simulink model "foc_demo"  (R2021b)
settings: Solver=VariableStepAuto  StartTime=0.0  StopTime=1.0  RelTol=1e-3
undefined symbols (not defined in the file): Ki_cd, Ki_cq, Ki_w, Kp_cd, Kp_cq, Kp_w
libraries: slpidlib x3, spsDCVoltageSourceLib x1, spsPermanentMagnetSynchronousMachineLib x1, simulink x1, spsUniversalBridgeLib x1, spspowerguiLib x1
settings Model: SimulationMode=accelerator  Creator=Jiaxin Qian  LastModifiedBy=Jiaxin Qian

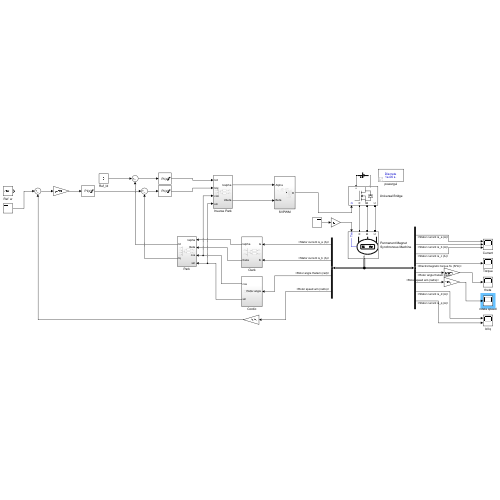
[thumbnail: Simulink's stored preview of the top-level diagram]
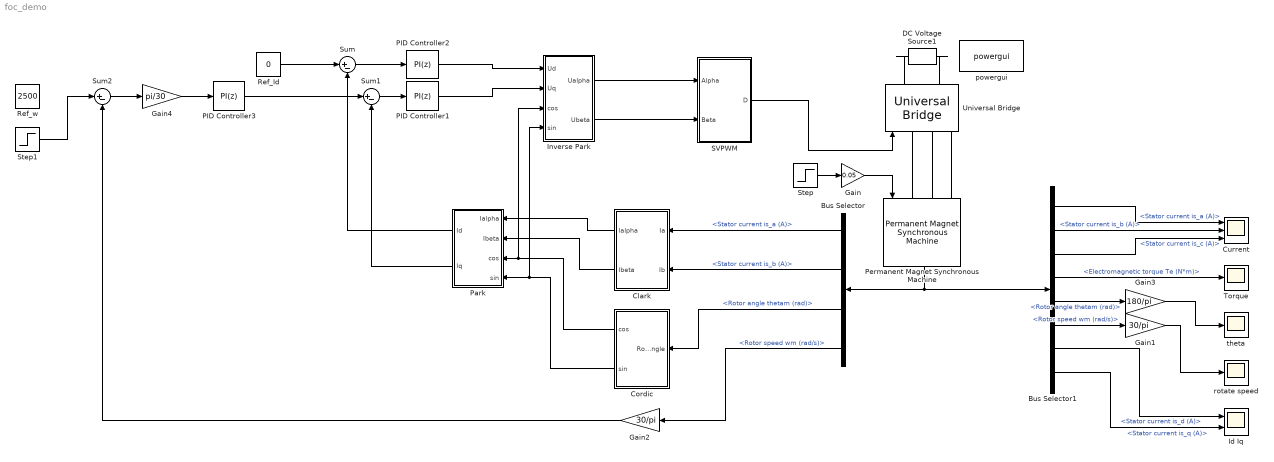
== system foc_demo ==
  Bus Selector : BusSelector  OutputSignals=Stator current is_a (A),Stator current is_b (A),Rotor angle thetam (rad),Rotor speed wm (rad/s)
  Bus Selector1 : BusSelector  OutputSignals=Stator current is_a (A),Stator current is_b (A),Stator current is_c (A),Electromagnetic torque Te (N*m),Rotor angle thetam (rad),Rotor speed wm (rad/s),Stator current is_d (A),Stator current is_q (A)
  Clark : Subsystem
  Cordic : Subsystem
  Current : Scope  NumInputPorts=3
  DC Voltage Source1 : spsDCVoltageSourceLib/DC Voltage Source  Amplitude=48  Measurements=None
  Gain : Gain  Gain=0.05
  Gain1 : Gain  Gain=30/pi
  Gain2 : Gain  Gain=30/pi
  Gain3 : Gain  Gain=180/pi
  Gain4 : Gain  Gain=pi/30
  Id Iq : Scope  NumInputPorts=2
  Inverse Park : Subsystem
  PID Controller1 : slpidlib/PID Controller  Controller=PI  Form=Parallel  TimeDomain=Discrete-time  UseExternalTs=off  SampleTime=-1  IntegratorMethod=Forward Euler  FilterMethod=Forward Euler  ControllerParametersSource=internal  P=Kp_cq  I=Ki_cq  D=0  UseFilter=on  N=100  TunerSelectOption=Transfer Function Based (PID Tuner App)  InitialConditionSource=internal  InitialConditionForIntegrator=0  InitialConditionForFilter=0  DifferentiatorICPrevScaledInput=0  ExternalReset=none  TrackingMode=off  Kt=1  LimitOutput=on  SatLimitsSource=internal  UpperSaturationLimit=29  LowerSaturationLimit=-29  LinearizeAsGain=on  AntiWindupMode=clamping  Kb=1  POutMin=[]  POutMax=[]  IOutMin=[]  IOutMax=[]  DOutMin=[]  DOutMax=[]  NOutMin=[]  NOutMax=[]  SumOutMin=[]  SumOutMax=[]  SaturationOutMin=[]  SaturationOutMax=[]  PParamMin=[]  PParamMax=[]  IParamMin=[]  IParamMax=[]  DParamMin=[]  DParamMax=[]  NParamMin=[]  NParamMax=[]  KbParamMin=[]  KbParamMax=[]  KtParamMin=[]  KtParamMax=[]  KbOutMin=[]  KbOutMax=[]  KtOutMin=[]  KtOutMax=[]  IntegratorOutMin=[]  IntegratorOutMax=[]  FilterOutMin=[]  FilterOutMax=[]  SumI1OutMin=[]  SumI1OutMax=[]  SumI2OutMin=[]  SumI2OutMax=[]  SumI3OutMin=[]  SumI3OutMax=[]  SumI4OutMin=[]  SumI4OutMax=[]  SumDOutMin=[]  SumDOutMax=[]  DifferentiatorOutMin=[]  DifferentiatorOutMax=[]  FilterDiffOutCoefMin=[]  FilterDiffOutCoefMax=[]  ReciprocalOutMin=[]  ReciprocalOutMax=[]  SumDenOutMin=[]  SumDenOutMax=[]  SumNumOutMin=[]  SumNumOutMax=[]  DivideOutMin=[]  DivideOutMax=[]  UdiffTsProdOutMin=[]  UdiffTsProdOutMax=[]  NTsProdOutMin=[]  NTsProdOutMax=[]  UintegralTsProdOutMin=[]  UintegralTsProdOutMax=[]  UngainTsProdOutMin=[]  UngainTsProdOutMax=[]  IntegratorContinuousStateAttributes=''  IntegratorStateMustResolveToSignalObject=off  IntegratorRTWStateStorageClass=Auto  FilterContinuousStateAttributes=''  FilterStateMustResolveToSignalObject=off  FilterRTWStateStorageClass=Auto  ParallelPVariant=InternalParameters  IdealPVariant=Disabled  IVariant=InternalParameters  DVariant=Disabled  IntegratorVariant=Discrete  SatVariant=Enabled  AWVariant=DiscClampingParallel  PCopyVariant=Disabled  TRVariant=Disabled  FdbkBlocksVariant=Forward  IdealPFdbkVariant=Disabled  SatFdbkVariant=Disabled  DerivativeFilterVariant=Disabled  NVariant=Disabled  NCopyVariant=Disabled_SignalSpec  FilterICVariant=Disabled  IntegratorICVariant=InternalICs  ExternalResetVariant=Disabled  TRSumVariant=Passthrough  SumFdbkVariant=Disabled  SumVariant=Sum_PI  TsampFilterVariant=InternalTs  TsampNgainVariant=Passthrough  TsampIntegralVariant=Passthrough  ExternalSaturationOutDataTypeStr=Inherit: Same as second input
  PID Controller2 : slpidlib/PID Controller  Controller=PI  Form=Parallel  TimeDomain=Discrete-time  UseExternalTs=off  SampleTime=-1  IntegratorMethod=Forward Euler  FilterMethod=Forward Euler  ControllerParametersSource=internal  P=Kp_cd  I=Ki_cd  D=0  UseFilter=on  N=100  TunerSelectOption=Transfer Function Based (PID Tuner App)  InitialConditionSource=internal  InitialConditionForIntegrator=0  InitialConditionForFilter=0  DifferentiatorICPrevScaledInput=0  ExternalReset=none  TrackingMode=off  Kt=1  LimitOutput=on  SatLimitsSource=internal  UpperSaturationLimit=29  LowerSaturationLimit=-29  LinearizeAsGain=on  AntiWindupMode=clamping  Kb=1  POutMin=[]  POutMax=[]  IOutMin=[]  IOutMax=[]  DOutMin=[]  DOutMax=[]  NOutMin=[]  NOutMax=[]  SumOutMin=[]  SumOutMax=[]  SaturationOutMin=[]  SaturationOutMax=[]  PParamMin=[]  PParamMax=[]  IParamMin=[]  IParamMax=[]  DParamMin=[]  DParamMax=[]  NParamMin=[]  NParamMax=[]  KbParamMin=[]  KbParamMax=[]  KtParamMin=[]  KtParamMax=[]  KbOutMin=[]  KbOutMax=[]  KtOutMin=[]  KtOutMax=[]  IntegratorOutMin=[]  IntegratorOutMax=[]  FilterOutMin=[]  FilterOutMax=[]  SumI1OutMin=[]  SumI1OutMax=[]  SumI2OutMin=[]  SumI2OutMax=[]  SumI3OutMin=[]  SumI3OutMax=[]  SumI4OutMin=[]  SumI4OutMax=[]  SumDOutMin=[]  SumDOutMax=[]  DifferentiatorOutMin=[]  DifferentiatorOutMax=[]  FilterDiffOutCoefMin=[]  FilterDiffOutCoefMax=[]  ReciprocalOutMin=[]  ReciprocalOutMax=[]  SumDenOutMin=[]  SumDenOutMax=[]  SumNumOutMin=[]  SumNumOutMax=[]  DivideOutMin=[]  DivideOutMax=[]  UdiffTsProdOutMin=[]  UdiffTsProdOutMax=[]  NTsProdOutMin=[]  NTsProdOutMax=[]  UintegralTsProdOutMin=[]  UintegralTsProdOutMax=[]  UngainTsProdOutMin=[]  UngainTsProdOutMax=[]  IntegratorContinuousStateAttributes=''  IntegratorStateMustResolveToSignalObject=off  IntegratorRTWStateStorageClass=Auto  FilterContinuousStateAttributes=''  FilterStateMustResolveToSignalObject=off  FilterRTWStateStorageClass=Auto  ParallelPVariant=InternalParameters  IdealPVariant=Disabled  IVariant=InternalParameters  DVariant=Disabled  IntegratorVariant=Discrete  SatVariant=Enabled  AWVariant=DiscClampingParallel  PCopyVariant=Disabled  TRVariant=Disabled  FdbkBlocksVariant=Forward  IdealPFdbkVariant=Disabled  SatFdbkVariant=Disabled  DerivativeFilterVariant=Disabled  NVariant=Disabled  NCopyVariant=Disabled_SignalSpec  FilterICVariant=Disabled  IntegratorICVariant=InternalICs  ExternalResetVariant=Disabled  TRSumVariant=Passthrough  SumFdbkVariant=Disabled  SumVariant=Sum_PI  TsampFilterVariant=InternalTs  TsampNgainVariant=Passthrough  TsampIntegralVariant=Passthrough  ExternalSaturationOutDataTypeStr=Inherit: Same as second input
  PID Controller3 : slpidlib/PID Controller  Controller=PI  Form=Parallel  TimeDomain=Discrete-time  UseExternalTs=off  SampleTime=-1  IntegratorMethod=Forward Euler  FilterMethod=Forward Euler  ControllerParametersSource=internal  P=Kp_w  I=Ki_w  D=0  UseFilter=on  N=100  TunerSelectOption=Transfer Function Based (PID Tuner App)  InitialConditionSource=internal  InitialConditionForIntegrator=0  InitialConditionForFilter=0  DifferentiatorICPrevScaledInput=0  ExternalReset=none  TrackingMode=off  Kt=1  LimitOutput=on  SatLimitsSource=internal  UpperSaturationLimit=5  LowerSaturationLimit=-5  LinearizeAsGain=on  AntiWindupMode=clamping  Kb=1  POutMin=[]  POutMax=[]  IOutMin=[]  IOutMax=[]  DOutMin=[]  DOutMax=[]  NOutMin=[]  NOutMax=[]  SumOutMin=[]  SumOutMax=[]  SaturationOutMin=[]  SaturationOutMax=[]  PParamMin=[]  PParamMax=[]  IParamMin=[]  IParamMax=[]  DParamMin=[]  DParamMax=[]  NParamMin=[]  NParamMax=[]  KbParamMin=[]  KbParamMax=[]  KtParamMin=[]  KtParamMax=[]  KbOutMin=[]  KbOutMax=[]  KtOutMin=[]  KtOutMax=[]  IntegratorOutMin=[]  IntegratorOutMax=[]  FilterOutMin=[]  FilterOutMax=[]  SumI1OutMin=[]  SumI1OutMax=[]  SumI2OutMin=[]  SumI2OutMax=[]  SumI3OutMin=[]  SumI3OutMax=[]  SumI4OutMin=[]  SumI4OutMax=[]  SumDOutMin=[]  SumDOutMax=[]  DifferentiatorOutMin=[]  DifferentiatorOutMax=[]  FilterDiffOutCoefMin=[]  FilterDiffOutCoefMax=[]  ReciprocalOutMin=[]  ReciprocalOutMax=[]  SumDenOutMin=[]  SumDenOutMax=[]  SumNumOutMin=[]  SumNumOutMax=[]  DivideOutMin=[]  DivideOutMax=[]  UdiffTsProdOutMin=[]  UdiffTsProdOutMax=[]  NTsProdOutMin=[]  NTsProdOutMax=[]  UintegralTsProdOutMin=[]  UintegralTsProdOutMax=[]  UngainTsProdOutMin=[]  UngainTsProdOutMax=[]  IntegratorContinuousStateAttributes=''  IntegratorStateMustResolveToSignalObject=off  IntegratorRTWStateStorageClass=Auto  FilterContinuousStateAttributes=''  FilterStateMustResolveToSignalObject=off  FilterRTWStateStorageClass=Auto  ParallelPVariant=InternalParameters  IdealPVariant=Disabled  IVariant=InternalParameters  DVariant=Disabled  IntegratorVariant=Discrete  SatVariant=Enabled  AWVariant=DiscClampingParallel  PCopyVariant=Disabled  TRVariant=Disabled  FdbkBlocksVariant=Forward  IdealPFdbkVariant=Disabled  SatFdbkVariant=Disabled  DerivativeFilterVariant=Disabled  NVariant=Disabled  NCopyVariant=Disabled_SignalSpec  FilterICVariant=Disabled  IntegratorICVariant=InternalICs  ExternalResetVariant=Disabled  TRSumVariant=Passthrough  SumFdbkVariant=Disabled  SumVariant=Sum_PI  TsampFilterVariant=InternalTs  TsampNgainVariant=Passthrough  TsampIntegralVariant=Passthrough  ExternalSaturationOutDataTypeStr=Inherit: Same as second input
  Park : Subsystem
  Permanent Magnet Synchronous Machine : spsPermanentMagnetSynchronousMachineLib/Permanent Magnet Synchronous Machine  NbPhases=3  FluxDistribution=Sinusoidal  RotorType=Round  MechanicalLoad=Torque Tm  PresetModel=No  ShowDetailedParameters=on  MeasurementBus=off  Resistance=0.75  Inductance=8.5e-3  dqInductances=[0.00095 0.00095]  La=0.00095  MachineConstant=Flux linkage established by magnets (V.s)  Flux=0.0103709  VoltageCst=9.4054  TorqueCst=0.077782  Flat=120  Mechanical=[3.3e-06 0 5]  PolePairs=4  InitialConditions=[0 0 0,0]  InitialConditions5ph=[0 0 0 0 0 0]  RefAngle=Aligned with phase A axis (original Park)  IterativeDiscreteModel=Trapezoidal non iterative  TsBlock=-1  TsPowergui=0
  Ref_Id : Constant  Value=0
  Ref_w : Constant  Value=2500
  SVPWM : Subsystem
  Step : Step  Time=0.25  SampleTime=0
  Step1 : Step  Time=0.5  Before=2500  After=-2500  SampleTime=0
  Sum : Sum  Inputs=|+-
  Sum1 : Sum  Inputs=|+-
  Sum2 : Sum  Inputs=|+-
  Torque : Scope
  Universal Bridge : spsUniversalBridgeLib/Universal Bridge  Arms=3  SnubberResistance=1e5  SnubberCapacitance=inf  Device=MOSFET / Diodes  Ron=1e-3  Lon=0  ForwardVoltages="[  0  0  ]"  ForwardVoltage=0  GTOparameters=[ 10e-6 , 20e-6 ]  IGBTparameters=[ 1e-6 , 2e-6 ]  Measurements=None  Measurements_2=None  converterType=Rectifier
  powergui : spspowerguiLib/powergui  Priority=1  SimulationMode=Discrete  SampleTime=1e-6  frequency=60  Iterations=50  frequencyindice=0  Pbase=100e6  ErrMax=1e-4  UnitsV=kV  UnitsW=MW  buscounter=0  FunctionMessages=off  echomessages=off  EnableUseOfTLC=off  CurrentSourceSwitches=off  DisableSnubberDevices=off  DisableRonSwitches=off  DisableVfSwitches=off  DisplayEquations=off  AutomaticDiscreteSolvers=off  SolverType=Tustin/Backward Euler (TBE)  Interpol=off  ExternalGateDelay=off  methode=off  Ts=100  x0status=blocks  SPID=on  SwTol=0  HookPort=off  NonlinearTolerance=1e-4  nMaxIteration=100  ContinueOnMaxIteration=off  RestoreLinks=warning  ResistiveCurrentMeasurement=off  Frange=[0:2:500]  Ylog=off  Xlog=on  ShowGrid=off  save=off  variable=ZData  structure=0  ZoomFFT=off  StartTime=0.0  cycles=1  DisplayStyle=1  fundamental=60  FreqAxis=off  MaxFrequency=1000  frequencyindicesteady=1  RmsSteady=1  display=off
  rotate speed : Scope
  theta : Scope
  wires:
  Permanent Magnet Synchronous Machine/1 -> Bus Selector1/1, Bus Selector/1
  Bus Selector1/4 -> Torque/1  "<Electromagnetic torque Te (N*m)>"
  Bus Selector1/1 -> Current/1  "<Stator current is_a (A)>"
  Bus Selector1/2 -> Current/2  "<Stator current is_b (A)>"
  Bus Selector1/3 -> Current/3  "<Stator current is_c (A)>"
  Sum/1 -> PID Controller2/1
  Sum1/1 -> PID Controller1/1
  Ref_Id/1 -> Sum/1
  Bus Selector1/5 -> Gain3/1  "<Rotor angle thetam (rad)>"
  Bus Selector1/6 -> Gain1/1  "<Rotor speed wm (rad/s)>"
  Gain1/1 -> rotate speed/1
  Gain3/1 -> theta/1
  SVPWM/1(D) -> Universal Bridge/1
  Clark/1(Ialpha) -> Park/1(Ialpha)
  Clark/2(Ibeta) -> Park/2(Ibeta)
  Park/1(Id) -> Sum/2
  Park/2(Iq) -> Sum1/2
  Inverse Park/1(Ualpha) -> SVPWM/1(Alpha)
  Inverse Park/2(Ubeta) -> SVPWM/2(Beta)
  Cordic/1(cos) -> Park/3(cos), Inverse Park/3(cos)
  Cordic/2(sin) -> Park/4(sin), Inverse Park/4(sin)
  Bus Selector/3 -> Cordic/1(Rotor angle)  "<Rotor angle thetam (rad)>"
  Bus Selector/1 -> Clark/1(Ia)  "<Stator current is_a (A)>"
  Bus Selector/2 -> Clark/2(Ib)  "<Stator current is_b (A)>"
  Bus Selector1/7 -> Id Iq/1  "<Stator current is_d (A)>"
  Bus Selector1/8 -> Id Iq/2  "<Stator current is_q (A)>"
  Bus Selector/4 -> Gain2/1  "<Rotor speed wm (rad/s)>"
  Sum2/1 -> Gain4/1
  PID Controller3/1 -> Sum1/1
  Gain2/1 -> Sum2/2
  Step/1 -> Gain/1
  Gain/1 -> Permanent Magnet Synchronous Machine/1
  PID Controller2/1 -> Inverse Park/1(Ud)
  PID Controller1/1 -> Inverse Park/2(Uq)
  Gain4/1 -> PID Controller3/1
  Step1/1 -> Sum2/1
  connections:
  Universal Bridge/LConn1 -- Permanent Magnet Synchronous Machine/LConn1
  Universal Bridge/LConn2 -- Permanent Magnet Synchronous Machine/LConn2
  Universal Bridge/LConn3 -- Permanent Magnet Synchronous Machine/LConn3
  DC Voltage Source1/RConn1 -- Universal Bridge/RConn1
  DC Voltage Source1/LConn1 -- Universal Bridge/RConn2

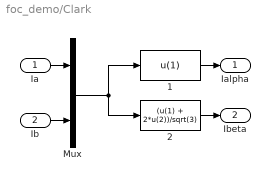
== system foc_demo/Clark ==
  Ia : Inport
  Ib : Inport  Port=2
  1 : Fcn  Expr=u(1)
  2 : Fcn  Expr=(u(1) + 2*u(2))/sqrt(3)
  Mux : Mux  Inputs=2
  Ialpha : Outport
  Ibeta : Outport  Port=2
  wires:
  Mux/1 -> 1/1, 2/1
  2/1 -> Ibeta/1
  Ia/1 -> Mux/1
  1/1 -> Ialpha/1
  Ib/1 -> Mux/2

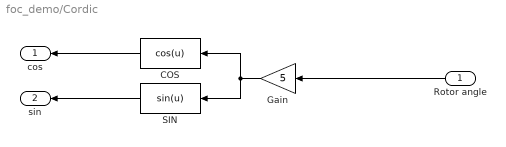
== system foc_demo/Cordic ==
  Rotor angle : Inport
  COS : Fcn  Expr=cos(u)
  Gain : Gain  Gain=5
  SIN : Fcn  Expr=sin(u)
  cos : Outport
  sin : Outport  Port=2
  wires:
  Gain/1 -> COS/1, SIN/1
  Rotor angle/1 -> Gain/1
  COS/1 -> cos/1
  SIN/1 -> sin/1

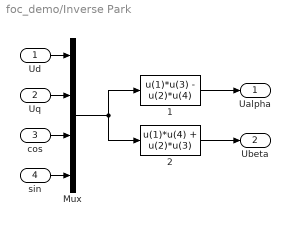
== system foc_demo/Inverse Park ==
  Ud : Inport
  Uq : Inport  Port=2
  cos : Inport  Port=3
  sin : Inport  Port=4
  1 : Fcn  Expr=u(1)*u(3) - u(2)*u(4)
  2 : Fcn  Expr=u(1)*u(4) + u(2)*u(3)
  Mux : Mux
  Ualpha : Outport
  Ubeta : Outport  Port=2
  wires:
  cos/1 -> Mux/3
  sin/1 -> Mux/4
  Mux/1 -> 2/1, 1/1
  2/1 -> Ubeta/1
  Ud/1 -> Mux/1
  1/1 -> Ualpha/1
  Uq/1 -> Mux/2

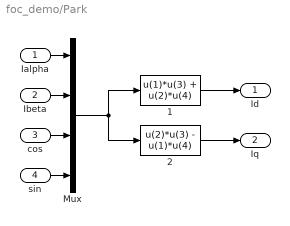
== system foc_demo/Park ==
  Ialpha : Inport
  Ibeta : Inport  Port=2
  cos : Inport  Port=3
  sin : Inport  Port=4
  1 : Fcn  Expr=u(1)*u(3) + u(2)*u(4)
  2 : Fcn  Expr=u(2)*u(3) - u(1)*u(4)
  Mux : Mux
  Id : Outport
  Iq : Outport  Port=2
  wires:
  Ibeta/1 -> Mux/2
  1/1 -> Id/1
  Ialpha/1 -> Mux/1
  2/1 -> Iq/1
  Mux/1 -> 1/1, 2/1
  sin/1 -> Mux/4
  cos/1 -> Mux/3

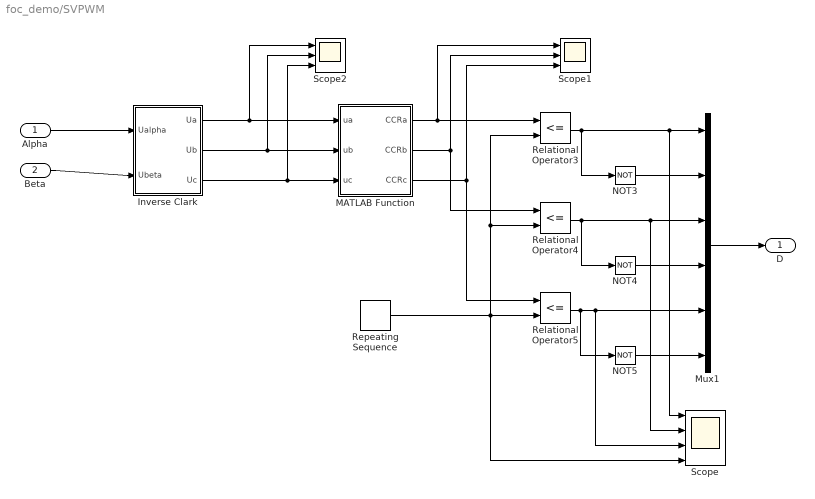
== system foc_demo/SVPWM ==
  Alpha : Inport
  Beta : Inport  Port=2
  Inverse Clark : Subsystem
  MATLAB Function : MATLAB Function  TreatAsAtomicUnit=on
  Mux1 : Mux  Inputs=6
  NOT3 : Logic  Operator=NOT  IconShape=distinctive  AllPortsSameDT=off  OutDataTypeStr=boolean
  NOT4 : Logic  Operator=NOT  IconShape=distinctive  AllPortsSameDT=off  OutDataTypeStr=boolean
  NOT5 : Logic  Operator=NOT  IconShape=distinctive  AllPortsSameDT=off  OutDataTypeStr=boolean
  Relational Operator3 : RelationalOperator  Operator=<=  OutDataTypeStr=boolean  RndMeth=Simplest
  Relational Operator4 : RelationalOperator  Operator=<=  OutDataTypeStr=boolean  RndMeth=Simplest
  Relational Operator5 : RelationalOperator  Operator=<=  OutDataTypeStr=boolean  RndMeth=Simplest
  Repeating Sequence : simulink/Sources/Repeating Sequence  rep_seq_t=[0 1/40000 1/20000]  rep_seq_y=[0 24 0]
  Scope : Scope  NumInputPorts=4
  Scope1 : Scope  NumInputPorts=3
  Scope2 : Scope  NumInputPorts=3
  D : Outport  VectorParamsAs1DForOutWhenUnconnected=off
  wires:
  Repeating Sequence/1 -> Scope/4, Relational Operator5/2, Relational Operator4/2, Relational Operator3/2
  Relational Operator3/1 -> NOT3/1, Scope/1, Mux1/1
  NOT3/1 -> Mux1/2
  Relational Operator4/1 -> NOT4/1, Scope/2, Mux1/3
  NOT4/1 -> Mux1/4
  Relational Operator5/1 -> Scope/3, Mux1/5, NOT5/1
  NOT5/1 -> Mux1/6
  Mux1/1 -> D/1
  MATLAB Function/1(CCRa) -> Scope1/1, Relational Operator3/1
  MATLAB Function/2(CCRb) -> Relational Operator4/1, Scope1/2
  MATLAB Function/3(CCRc) -> Relational Operator5/1, Scope1/3
  Inverse Clark/2(Ub) -> Scope2/2, MATLAB Function/2(ub)
  Inverse Clark/3(Uc) -> Scope2/3, MATLAB Function/3(uc)
  Inverse Clark/1(Ua) -> Scope2/1, MATLAB Function/1(ua)
  Alpha/1 -> Inverse Clark/1(Ualpha)
  Beta/1 -> Inverse Clark/2(Ubeta)

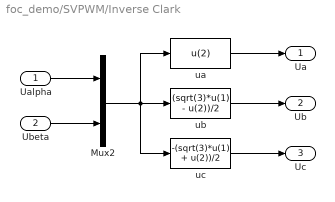
== system foc_demo/SVPWM/Inverse Clark ==
  Ualpha : Inport
  Ubeta : Inport  Port=2
  Mux2 : Mux  Inputs=2
  ua : Fcn  Expr=u(2)
  ub : Fcn  Expr=(sqrt(3)*u(1) - u(2))/2
  uc : Fcn  Expr=-(sqrt(3)*u(1) + u(2))/2
  Ua : Outport
  Ub : Outport  Port=2
  Uc : Outport  Port=3
  wires:
  Ualpha/1 -> Mux2/1
  Ubeta/1 -> Mux2/2
  Mux2/1 -> uc/1, ub/1, ua/1
  ub/1 -> Ub/1
  uc/1 -> Uc/1
  ua/1 -> Ua/1

== matlab function foc_demo/SVPWM/MATLAB Function ==
  data: ua input; CCRa output; ub input; uc input; CCRb output; CCRc output
function [CCRa,CCRb,CCRc] = SVPWM(ua,ub,uc)
    sector = SVPWM_Select_Sector(ua,ub,uc);
    [CCRa,CCRb,CCRc] = SVPWM_Calculate_Workingtime(sector,ua,ub,uc);
end

function sector = SVPWM_Select_Sector(ua,ub,uc)
    if ua>0
        A = 1;
    else
        A = 0;
    end
    if ub>0
        B = 1;
    else
        B = 0;
    end
    if uc>0
        C = 1;
    else
        C = 0;
    end

    switch A + 2*B + 4*C
        case 1
            sector = 2;
        case 2
            sector = 6;
        case 3
            sector = 1;
        case 4
            sector = 4;
        case 5
            sector = 3;
        case 6
            sector = 5;
        otherwise
            sector = 1;
    end
end

function [CCRa,CCRb,CCRc] = SVPWM_Calculate_Workingtime(sector,ua,ub,uc)
    Udc = 48;
    switch sector
        case 1
            tx = ub;
            ty = ua;
            CCRa = (Udc - tx - ty)/4;
            CCRb = (Udc + tx - ty)/4;
            CCRc = (Udc + tx + ty)/4;
        case 2
            tx = -ub;
            ty = -uc;
            CCRa = (Udc + tx - ty)/4;
            CCRb = (Udc - tx - ty)/4;
            CCRc = (Udc + tx + ty)/4;
        case 3
            tx = ua;
            ty = uc;
            CCRa = (Udc + tx + ty)/4;
            CCRb = (Udc - tx - ty)/4;
            CCRc = (Udc + tx - ty)/4;
        case 4
            tx = -ua;
            ty = -ub;
            CCRa = (Udc + tx + ty)/4;
            CCRb = (Udc + tx - ty)/4;
            CCRc = (Udc - tx - ty)/4;
        case 5
            tx = uc;
            ty = ub;
            CCRa = (Udc + tx - ty)/4;
            CCRb = (Udc + tx + ty)/4;
            CCRc = (Udc - tx - ty)/4;
        case 6
            tx = -uc;
            ty = -ua;
            CCRa = (Udc - tx - ty)/4;
            CCRb = (Udc + tx + ty)/4;
            CCRc = (Udc + tx - ty)/4;
        otherwise
            tx = ub;
            ty = ua;
            CCRa = (Udc - tx - ty)/4;
            CCRb = (Udc + tx - ty)/4;
            CCRc = (Udc + tx + ty)/4;
    end
    
end
